simulink library "Adaptive_library"  (R2016b)
settings: Solver=ode45  StartTime=0.0  StopTime=10.0  RelTol=1e-3  EnableMultiTasking=on
undefined symbols (not defined in the file or in its folder): functionType
libraries: Adaptive_library x7, vrlib x2, dspinverses x2
settings Model: Creator=jinkale  LastModifiedBy=dell
settings DataIOCC: LimitDataPoints=on  SaveFormat=Array
settings OptimizationCC: LifeSpan=inf
settings DebuggingCC: SFUnexpectedBacktrackingDiag=warning  SFNoUnconditionalDefaultTransitionDiag=warning  SFExecutionAtInitializationDiag=none
settings HardwareCC: ProdBitPerPointer=32  ProdBitPerSizeT=32  ProdBitPerPtrDiffT=32  ProdLargestAtomicFloat=None  ProdIntDivRoundTo=Undefined  ProdEndianess=Unspecified  ProdWordSize=32  ProdHWDeviceType=32-bit Generic
settings ModelReferenceCC: PropagateSignalLabelsOutOfModel=off
settings GRTTargetCC: TargetLangStandard=C89/C90 (ANSI)  GeneratePreprocessorConditionals=Disable all
settings ConfigComp: CovMetricSettings=dw  CovHtmlReporting=on  CovSaveCumulativeToWorkspaceVar=on  CovSaveSingleToWorkspaceVar=on  CovExternalEMLEnable=off

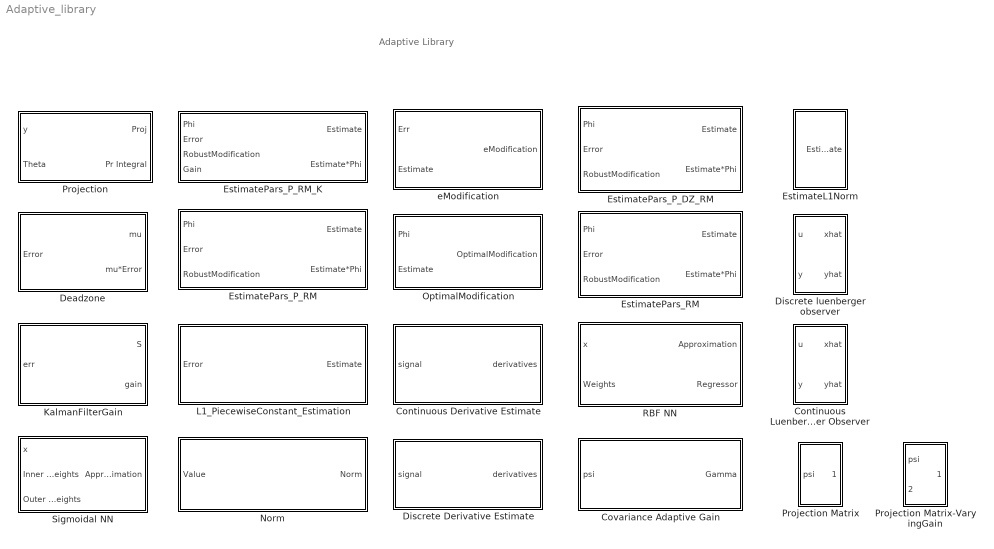
== system Adaptive_library ==
  note: Adaptive Library
  Continuous Derivative Estimate : Subsystem  mask{N=1, poles=[-300,-350], x0=0, satmax=10, satmin=-10}
      mask prompts: N "Derivative order"; poles "Observer poles"; x0 "Initial conditions"; satmax "Maximum saturation"; satmin "Minimum saturation"
      mask help:
      | % Name: Continuous Derivative Estimate
      | % Author: Alessio Russo - russo.alessio890@gmail.com
      | % Last update: 2/12/2016
      | % INPUTS
      | %      -signal: signal to differentiate
      | % OUTPUTS:
      | %      -derivatives: derivatives of signal
      |
      | Derivative order: up to which order we should estimate the derivative of signal
      | Observer poles: poles of the observer. Higher in absolute value-> faster. But there is peaking phenomena
      | Saturation: saturation on the signal derivatives
      mask init:
      | N=N+1;
      | A = [zeros(N-1,1), eye(N-1); zeros(1, N)];
      | B = zeros(N,1);
      | C = [1, zeros(1,N-1)];
      | D = 0;
      | 
      | L = place(A', C', poles)';
  "Continuous Luenberger Observer " : Subsystem  mask{A=0, B=0, C=0, D=0, L=0, x0=0, satmax=10, satmin=-10}
      mask prompts: L "Observer gain"; x0 "Initial condition"; satmax "Max saturation"; satmin "Min saturation"
      mask help:
      | % Name: Continuous Luenberger Observer
      | % Author: Alessio Russo - russo.alessio890@gmail.com
      | % Last update: 2/12/2016
      | % INPUTS
      | %      -u: input signal of the plant to observe
      | %      -y: output signal of the plant to observe
      | % OUTPUTS:
      | %      -xhat: estimated state of the plant
      | %      -yhat: estimated output of the plant
      |
      |
      | Continuous luenberger observer. The saturation block saturates the states.
      mask DialogControl Container3 Prompt: Parameters
  Covariance Adaptive Gain : Subsystem  mask{Gamma0=1, alpha1=1, alpha2=1, Kalpha1=1}
      mask prompts: Gamma0 "Initial condition"
      mask help:
      | % Name: Covariance Adaptive Gain
      | % Author: Alessio Russo - russo.alessio890@gmail.com
      | % Last update: 2/12/2016
      | % INPUTS
      | %      -psi: input feature psi(x)
      | % OUTPUTS:
      | %      -Gamma: adaptive gain
      |
      | Initial condition - Gamma0: positive definite diagonal matrix which defines the initial values for the adaptive gian.
      | Forgetting factor - Alpha1: positive definite diagonal matrix which defines the forgetting factor.
      | Excitation gain - Alpha2: positive definite diagonla matrix that defines the gain of the excitation
      | Maximum gain bound - Kalpha1 : defines the maximum bound of the inf norm of gamma
      |
      |
      | Equation:
      |
      | \dot{Gamma} = alpha1*Gamma- alpha2* Gamma*psi*psi^T *Gamma
      mask init:
      | if (Kalpha1 <= 0 || isscalar(Kalpha1)==0)
      |     error('Kalpha1 should be a scalar number greater than 0.')
      | end
      | 
      | if (isdiag(Gamma0)==0 || isdiag(alpha1)==0 || isdiag(alpha2)==0)
      |     error('One of the matrices is not diagonal.')
      | end
      | %the second value that chol returns is whether a matrix is positive
      | %definite (0) or not (1)
      | [~,p1] = chol(Gamma0);
      | [~,p2] = chol(alpha1);
      | [~,p3] = chol(alpha2);
      | 
      | if (p1 > 0)
      |     error('Gamma0 is not positive definite.')
      | end
      | if (p2 > 0)
      |     error('alpha1 is not positive definite')
      | end
      | 
      | if(p3 > 0)
      |     error('alpha2 is not positive definite')
      | end
  Deadzone : Subsystem  mask{delta=0.5, e0=1, Weight=1}
      mask prompts: delta "delta ( 0 < delta < 1)"; e0 "e0 ( e0 >0 )"
      mask help:
      | % Name: Deadzone with lipschitz modification
      | % Author: Alessio Russo - russo.alessio890@gmail.com
      | % Last update: 2/12/2016
      | % INPUTS
      | %      -Error: error between reference and plant
      | % OUTPUTS:
      | %      -mu: calculates mu(||Error||)
      | %      -mu*Error: claculates mu(||Error||)*Error
      |
      |
      | Implements the lipschitz-continuous version of the deadzone.
      |
      | mu(Error) = max(0, min (1, (||Error|- delta*e0)/((1-delta)*e0)));
      |
      | 0 < delta < 1
      | e0 > 0
      mask init:
      | if (e0<=0)
      |     error('e0 should be  greater than 0.')
      | end
      | 
      | if (delta <= 0 || delta >= 1)
      |     error('delta should lay in (0,1).');
      | end
  Discrete Derivative Estimate : Subsystem  mask{N=1, poles=[0.05,0.01], x0=0, ts=0.01, satmax=10, satmin=-10}
      mask prompts: N "Derivative order"; poles "Observer poles"; x0 "Initial conditions"; ts "Sampling time"; satmax "Maximum saturation"; satmin "Minimum saturation"
      mask help:
      | % Name: Discrete  Derivative Estimate
      | % Author: Alessio Russo - russo.alessio890@gmail.com
      | % Last update: 2/12/2016
      | % INPUTS
      | %      -signal: signal to differentiate
      | % OUTPUTS:
      | %      -derivatives: derivatives of signal
      |
      | Derivative order: up to which order we should estimate the derivative of signal
      | Observer poles: poles of the observer. Lower in absolute value-> faster. But there is peaking phenomena
      | Saturation: saturation on the signal derivatives
      mask init:
      | N=N+1;
      | A = [zeros(N-1,1), eye(N-1); zeros(1, N)];
      | B = zeros(N,1);
      | C = [1, zeros(1,N-1)];
      | D = 0;
      | 
      | A = (eye(N)+0.5*A*ts)*inv(eye(N)-0.5*A*ts);
      | L = place(A', C', poles)';
  Discrete luenberger observer : Subsystem  mask{A=0, B=0, C=0, D=0, L=0, x0=0, ts=0.1, satmax=10, satmin=-10}
      mask prompts: L "Observer gain"; x0 "Initial condition"; ts "Sampling time"; satmax "Maximum saturation"; satmin "Minimum saturation"
      mask help:
      | % Name: Discrete Luenberger Observer
      | % Author: Alessio Russo - russo.alessio890@gmail.com
      | % Last update: 2/12/2016
      | % INPUTS
      | %      -u: input signal of the plant to observe
      | %      -y: output signal of the plant to observe
      | % OUTPUTS:
      | %      -xhat: estimated state of the plant
      | %      -yhat: estimated output of the plant
      |
      |
      | Discrete luenberger observer. The saturation block saturates the states.
  EstimateL1Norm : Subsystem  mask{A=0, B=0, C=0, D=0, x0=0, df=100}
      mask prompts: x0 "X0 (Initial conditions)"; df "Derivative Frequency"
      mask help:
      | % Name: EstimateL1Norm
      | % Author: Alessio Russo - russo.alessio890@gmail.com
      | % Last update: 2/12/2016
      |
      |
      | BLOCK NOT COMPLETED! The output should be the l1 norm estimate of a linear SISO system
  EstimatePars_P_DZ_RM : Subsystem  mask{Gamma=100, P=0, B=0, EpsilonTheta=0.1, Prmax=1, Center=0, Pr0=0, delta=0.5, e0=1}
      mask prompts: EpsilonTheta "Epsilon"; Prmax "Bound (radius of the ball)"; Center "Center (of the ball)"; Pr0 "Initialization of the integral"; delta "delta ( 0 < delta < 1)"; e0 "e0 ( e0 >0 )"
      mask help:
      | % Name: EstimatePars_P_DZ_RM
      | % Author: Alessio Russo - russo.alessio890@gmail.com
      | % Last update: 2/12/2016
      | % INPUTS
      | %      -Phi: input feature phi(x)
      | %      -Error: error signal
      | %      -RobustModification: any additive robust modification can be included in this port
      | % OUTPUTS:
      | %      -Estimate: uncertainty estimate
      | %      -Estimate*Phi: uncertainty times the input feature
      |
      |
      | Used in conjuction with the projection operator and the lipschitz version of the deadzone,
      | implemented as follows:
      |
      | mu(e) = max(0, min (1, (||e|- delta*e0)/((1-delta)*e0)));
      |
      | 0 < delta < 1
      | e0 > 0
      mask init:
      | Pb=P*B;
      | 
      | if (e0<=0)
      |     error('e0 should be  greater than 0.')
      | end
      | 
      | if (delta <= 0 || delta >= 1)
      |     error('delta should lay in (0,1).');
      | end
  EstimatePars_P_RM : Subsystem  mask{Gamma=1, P=0, B=0, EpsilonTheta=0.1, Prmax=1, Center=0, Pr0=0}
      mask prompts: EpsilonTheta "Epsilon"; Prmax "Bound (radius of the ball)"; Center "Center (of the ball)"; Pr0 "Initialization of the integral"
      mask help:
      | % Name: EstimatePars_P_RM
      | % Author: Alessio Russo - russo.alessio890@gmail.com
      | % Last update: 2/12/2016
      | % INPUTS
      | %      -Phi: input feature phi(x)
      | %      -Error: error signal
      | %      -RobustModification: any additive robust modification can be included in this port
      | % OUTPUTS:
      | %      -Estimate: uncertainty estimate
      | %      -Estimate*Phi: uncertainty times the input feature
      |
      | The block implements the projection operator
      mask init:
      | Pb=P*B;
  EstimatePars_P_RM_K : Subsystem  mask{P=0, B=0, EpsilonTheta=0.1, Prmax=1, Center=0, Pr0=0}
      mask prompts: EpsilonTheta "Epsilon"; Prmax "Bound (radius of the ball)"; Center "Center (of the ball)"; Pr0 "Initialization of the integral"
      mask help:
      | % Name: EstimatePars_P_RM_K
      | % Author: Alessio Russo - russo.alessio890@gmail.com
      | % Last update: 2/12/2016
      | % INPUTS
      | %      -Phi: input feature phi(x)
      | %      -Error: error signal
      | %      -RobustModification: any additive robust modification can be included in this port
      | %      -Gain: adaptive gain (external)
      | % OUTPUTS:
      | %      -Estimate: uncertainty estimate
      | %      -Estimate*Phi: uncertainty times the input feature
      |
      | The block implements the projection operator
      mask init:
      | Pb=P*B;
  EstimatePars_RM : Subsystem  mask{Gamma=0, x0=0, P=0, B=0}
      mask prompts: x0 "InitialValue"
      mask help:
      | % Name: EstimatePars_RM
      | % Author: Alessio Russo - russo.alessio890@gmail.com
      | % Last update: 2/12/2016
      | % INPUTS
      | %      -Phi: input feature phi(x)
      | %      -Error: error signal
      | %      -RobustModification: any additive robust modification can be included in this port
      | % OUTPUTS:
      | %      -Estimate: uncertainty estimate
      | %      -Estimate*Phi: uncertainty times the input feature
      mask init:
      | Pb=P*B;
  KalmanFilterGain : Subsystem  mask{Q=1, R=1, S0=1, sigma=1}
      mask help:
      | % Name:  KalmanFilterGain
      | % Author: Alessio Russo - russo.alessio890@gmail.com
      | % Last update: 2/12/2016
      | % INPUTS
      | %      -err: error signal
      | % OUTPUTS:
      | %      -S: matrix S(t) used to calculate the adaptive gain
      | %      -gain: adaptive gain Gamma
      |
      | Gamma is calculated as follows
      |
      | Gamma = S*inv(R)
      |
      | where \dot{S} = -sigma *||e|| *S*inv(R)*S+Q
      |
      | and, Q,R are symmetric positive definite matrices (fixed). S0 defines the initial condition of S(t).
  L1_PiecewiseConstant_Estimation : Subsystem  mask{Bm=1, Bum=0, Ts=1, Am=-1, gamma=1, x0=0, satmax=inf, satmin=-inf}
      mask prompts: Bm "Bm (Matched)"; Bum "Bum (Unmatched)"; Ts "Sampling Time"; Am "Am (reference matrix of dynamics)"; x0 "Initial Value"; satmax "Max Saturation"; satmin "Min Saturation"
      mask help:
      | % Name: L1 Piecewise-constant adaptive law
      | % Author: Alessio Russo - russo.alessio890@gmail.com
      | % Last update: 2/12/2016
      | % INPUTS
      | %      -error: error signal
      | % OUTPUTS:
      | %      -estimate: uncertainty estimate
      |
      | The output of the block is the estimate that needs to be cancelled.
      mask init:
      | if (Ts<=0)
      |     error('Sampling time should be  greater than 0.')
      | end
      | 
      | if (gamma<=0)
      |     error('Gamma should be  greater than 0.')
      | end
      | 
      | if (sum(real(eig(Am))>=0))
      |     error('Am should be Hurwitz.');
      | end
      | 
      | 
      | mu = exp(Am*Ts);
      | if (isscalar(Bm)==1 || (size(Bm,1)==size(Bm,2)))
      |     B=Bm;
      | else
      |     B = [Bm, Bum];
      | end
      | PHIinv = inv(inv(Am)* ( exp(Am*Ts)- eye(size(Am,1)))*B);
  Norm : Subsystem
      mask help:
      | % Name: Norm
      | % Author: Alessio Russo - russo.alessio890@gmail.com
      | % Last update: 2/12/2016
      | % INPUTS
      | %      -Value: vector input
      | % OUTPUTS:
      | %      -Norm: euclidean norm of Value
  OptimalModification : Subsystem  mask{sigma=1, P=0, B=0, Am=0}
      mask help:
      | % Name: optimal modification
      | % Author: Alessio Russo - russo.alessio890@gmail.com
      | % Last update: 2/12/2016
      | % INPUTS
      | %      -phi: phi(x) , input feature
      | %      -estimate: uncertainty estimate
      | % OUTPUTS:
      | %      -optimal modification: gives as output the optimal modification that should be added to the adaptive law
      mask init:
      | OptConst = B'*P*inv(Am)*B;
  Projection : Subsystem  mask{EpsilonTheta=0.3, Prmax=0.5, Center=0, Pr0=0.1}
      mask prompts: EpsilonTheta "Epsilon"; Prmax "Bound (radius of the ball)"; Center "Center (of the ball)"; Pr0 "Initialization of integral"
      mask help:
      | % Name: Projection Operator with center modification
      | % Author: Alessio Russo - russo.alessio890@gmail.com
      | % Last update: 2/12/2016
      | % INPUTS
      | %      -y: value to project
      | %      -theta: current value of the estimate
      | % OUTPUTS:
      | %      -Proj: calculates Proj(theta,y)
      | %      -Pr Integral: integrates Proj(theta;y)
      |
      | Computes projection of the signal and safely integrate it.
      | Works both for scalar and vector signals.
      | It considers the parameter set as a ball at the setted center and radius.
      |
      | Epsilon defines when the projection operator starts to operate.
      mask init:
      | Thetamax = (Prmax) / sqrt(EpsilonTheta+1);
  Projection Matrix : Subsystem  mask{Gamma=1}
      mask prompts: Gamma "Adaptive gain matrix"
      mask help:
      | % Name: Projection Matrix
      | % Author: Alessio Russo - russo.alessio890@gmail.com
      | % Last update: 26/12/2016
      | % INPUTS
      | %      -psi: input feature psi(x)
      | % OUTPUTS:
      | %      -Proj: projection matrix
      |
      | Outputs a matrix that projects any vector on the null space of psi. Gamma is a positive definite symmetric matrix.
      |
      | The matrix is calculated based on the following law
      |
      | I- A(A^TA)^(-1)A^T, where A = Gamma*psi
  Projection Matrix-VaryingGain : Subsystem
      mask help:
      | % Name: Projection Matrix-VaryingGain
      | % Author: Alessio Russo - russo.alessio890@gmail.com
      | % Last update: 26/12/2016
      | % INPUTS
      | %      -psi: input feature psi(x)
      | %      -Gamma: definite positive symmetric matrix
      | % OUTPUTS:
      | %      -Proj: projection matrix
      |
      | Outputs a matrix that projects any vector on the null space of psi. Gamma is a positive definite symmetric matrix.
      |
      | The matrix is calculated based on the following law
      |
      | I- A(A^TA)^(-1)A^T, where A = Gamma*psi
  RBF NN : Subsystem  mask{Mean=0, Variance=0}
      mask help:
      | % Name: RBF NN
      | % Author: Alessio Russo - russo.alessio890@gmail.com
      | % Last update: 2/12/2016
      | % INPUTS
      | %      -x: input feature
      | %      -Weights: weights of the GMM
      | % OUTPUTS:
      | %      -Approximation: output of the GMM NN
      | %      -Regressor: vector of the basis functions output
      |
      | This RBF block implement the GMM (gaussian mixture model) which is just a linear combination of gaussian functions.
      | Mean is  a vector containing the center of the gaussians functions. Variance is a vector defining
      | the variance of each gaussian.
      |
      | y(x) = W * [exp(-Variance * (x-Mean)^2)]
  Sigmoidal NN : Subsystem  mask{rf=Logistic sigmoid}
      mask prompts: rf "Ridge Function"
      mask help:
      | % Name: Sigmoidal NN
      | % Author: Alessio Russo - russo.alessio890@gmail.com
      | % Last update: 2/12/2016
      | % INPUTS
      | %      -x: input feature
      | %      -Inner Weights: weights matrix of the hidden layer
      | %      - Outer Weight: weights matrix of the output layer
      | % OUTPUTS:
      | %      -Approximation: output of the NN
      |
      | Sigmoidal NN. The logistic or hyperbolic tangent functions can be used
      mask init:
      | switch rf
      |     case 'Logistic sigmoid'
      |         FunctionType = -1;
      |     case 'Hyperbolic tangent'
      |         FunctionType = 1;
      | end
      mask TypeOptions rf: Logistic sigmoid | Hyperbolic tangent
  eModification : Subsystem  mask{sigma=0, P=0, B=0}
      mask help:
      | % Name: e modification
      | % Author: Alessio Russo - russo.alessio890@gmail.com
      | % Last update: 2/12/2016
      | % INPUTS
      | %      -err: error signal
      | %      -estimate: uncertainty estimate
      | % OUTPUTS:
      | %      -e modification: gives as output sigma*||e(t)^TPB||*estimate
      |
      | Givent the values for sigma, P, B calculates sigma*||e(t)^TPB||*estimate
      mask init:
      | Pb=P*B;

== system Adaptive_library/Continuous Derivative Estimate ==
  signal : Inport
  Continuous Luenberger Observer1 : Adaptive_library/Continuous Luenberger Observer  A=A  B=B  C=C  D=D  L=L  x0=x0  satmax=satmax  satmin=satmin
  Ground : Ground
  Terminator : Terminator
  derivatives : Outport
  wires:
  Continuous Luenberger Observer1/2 -> Terminator/1
  Continuous Luenberger Observer1/1 -> derivatives/1
  Ground/1 -> Continuous Luenberger Observer1/1
  signal/1 -> Continuous Luenberger Observer1/2

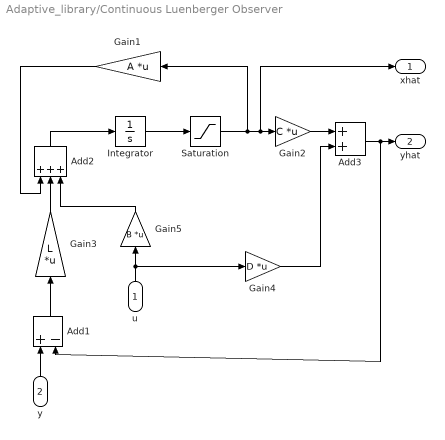
== system Adaptive_library/Continuous Luenberger Observer  ==
  u : Inport
  y : Inport  Port=2
  Add1 : Sum  Inputs=+-
  Add2 : Sum  Inputs=+++
  Add3 : Sum
  Gain1 : Gain  Gain=A  Multiplication=Matrix(K*u)
  Gain2 : Gain  Gain=C  Multiplication=Matrix(K*u)
  Gain3 : Gain  Gain=L  Multiplication=Matrix(K*u)
  Gain4 : Gain  Gain=D  Multiplication=Matrix(K*u)
  Gain5 : Gain  Gain=B  Multiplication=Matrix(K*u)
  Integrator : Integrator  InitialCondition=x0
  Saturation : Saturate  UpperLimit=satmax  LowerLimit=satmin
  xhat : Outport
  yhat : Outport  Port=2
  wires:
  Gain3/1 -> Add2/2
  Gain1/1 -> Add2/1
  Integrator/1 -> Saturation/1
  Add2/1 -> Integrator/1
  y/1 -> Add1/1
  Add1/1 -> Gain3/1
  Gain5/1 -> Add2/3
  Gain2/1 -> Add3/1
  Gain4/1 -> Add3/2
  u/1 -> Gain4/1, Gain5/1
  Add3/1 -> Add1/2, yhat/1
  Saturation/1 -> xhat/1, Gain2/1, Gain1/1

== system Adaptive_library/Covariance Adaptive Gain ==
  psi : Inport
  Integrator : Integrator  InitialCondition=Gamma0
  Math Function : Math  Operator=transpose  SaturateOnIntegerOverflow=on
  Math Function1 : Math  Operator=transpose  SaturateOnIntegerOverflow=on
  Product : Product  Multiplication=Matrix(*)
  Product1 : Product  Multiplication=Matrix(*)
  Subsystem : Subsystem
  Subtract : Sum  Inputs=+-
  alpha2 : Gain  Gain=alpha2  Multiplication=Matrix(K*u)
  Gamma : Outport
  wires:
  Math Function/1 -> Product/1
  Subtract/1 -> Integrator/1
  Integrator/1 -> Gamma/1, Product/2, Subsystem/1(Gamma)
  alpha2/1 -> Subtract/2
  Product/1 -> Product1/2, Math Function1/1
  psi/1 -> Math Function/1
  Math Function1/1 -> Product1/1
  Product1/1 -> alpha2/1
  Subsystem/1(alpha1*Gamma) -> Subtract/1

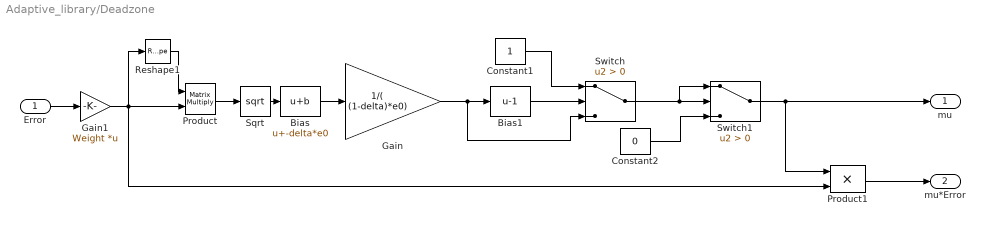
== system Adaptive_library/Deadzone ==
  Error : Inport
  Bias : Bias  Bias=-delta*e0
  Bias1 : Bias  Bias=-1
  Constant1 : Constant
  Constant2 : Constant  Value=0
  Gain : Gain  Gain=1/( (1-delta)*e0)
  Gain1 : Gain  Gain=Weight  Multiplication=Matrix(K*u)
  Product : Product  Multiplication=Matrix(*)
  Product1 : Product
  Reshape1 : Reshape  OutputDimensionality=Row vector (2-D)
  Sqrt : Sqrt  SaturateOnIntegerOverflow=on
  Switch : Switch  Criteria=u2 > Threshold
  Switch1 : Switch  Criteria=u2 > Threshold
  mu : Outport
  mu*Error : Outport  Port=2
  wires:
  Bias/1 -> Gain/1
  Gain/1 -> Switch/3, Bias1/1
  Bias1/1 -> Switch/2
  Constant1/1 -> Switch/1
  Switch/1 -> Switch1/1, Switch1/2
  Constant2/1 -> Switch1/3
  Switch1/1 -> Product1/1, mu/1
  Reshape1/1 -> Product/1
  Sqrt/1 -> Bias/1
  Product/1 -> Sqrt/1
  Product1/1 -> mu*Error/1
  Error/1 -> Gain1/1
  Gain1/1 -> Reshape1/1, Product1/2, Product/2

== system Adaptive_library/Discrete Derivative Estimate ==
  signal : Inport
  Discrete luenberger observer1 : Adaptive_library/Discrete luenberger observer  A=A  B=B  C=C  D=D  L=L  x0=x0  ts=ts  satmax=satmax  satmin=satmin
  Ground : Ground
  Terminator : Terminator
  Zero-Order Hold : ZeroOrderHold  SampleTime=ts
  Zero-Order Hold1 : ZeroOrderHold  SampleTime=ts
  derivatives : Outport
  wires:
  Discrete luenberger observer1/1 -> Zero-Order Hold1/1
  Ground/1 -> Discrete luenberger observer1/1
  signal/1 -> Zero-Order Hold/1
  Discrete luenberger observer1/2 -> Terminator/1
  Zero-Order Hold/1 -> Discrete luenberger observer1/2
  Zero-Order Hold1/1 -> derivatives/1

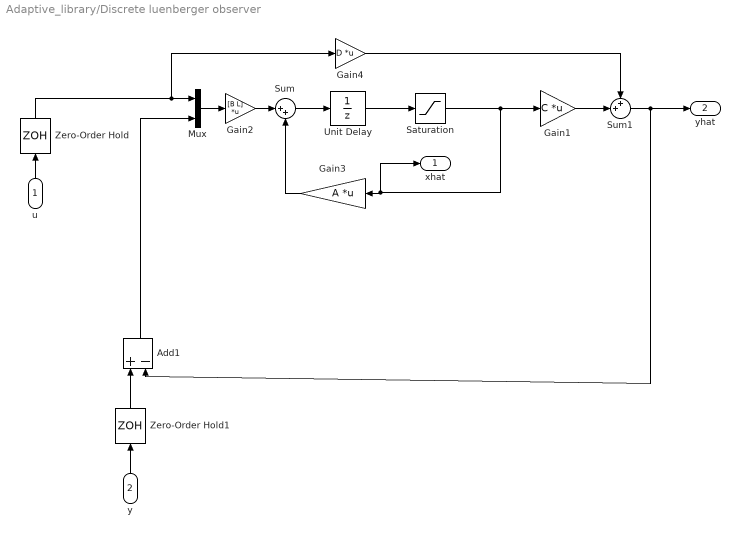
== system Adaptive_library/Discrete luenberger observer ==
  u : Inport
  y : Inport  Port=2
  Add1 : Sum  Inputs=+-
  Gain1 : Gain  Gain=C  Multiplication=Matrix(K*u)
  Gain2 : Gain  Gain=[B L]  Multiplication=Matrix(K*u)
  Gain3 : Gain  Gain=A  Multiplication=Matrix(K*u)
  Gain4 : Gain  Gain=D  Multiplication=Matrix(K*u)
  Mux : Mux  Inputs=2
  Saturation : Saturate  UpperLimit=satmax  LowerLimit=satmin
  Sum : Sum  Inputs=|++
  Sum1 : Sum  Inputs=++|
  Unit Delay : UnitDelay  InitialCondition=x0  SampleTime=ts
  Zero-Order Hold : ZeroOrderHold  SampleTime=ts
  Zero-Order Hold1 : ZeroOrderHold  SampleTime=ts
  xhat : Outport
  yhat : Outport  Port=2
  wires:
  Add1/1 -> Mux/2
  y/1 -> Zero-Order Hold1/1
  u/1 -> Zero-Order Hold/1
  Zero-Order Hold1/1 -> Add1/1
  Zero-Order Hold/1 -> Gain4/1, Mux/1
  Unit Delay/1 -> Saturation/1
  Mux/1 -> Gain2/1
  Gain2/1 -> Sum/1
  Sum/1 -> Unit Delay/1
  Gain3/1 -> Sum/2
  Gain1/1 -> Sum1/2
  Sum1/1 -> Add1/2, yhat/1
  Gain4/1 -> Sum1/1
  Saturation/1 -> Gain1/1, xhat/1, Gain3/1

== system Adaptive_library/EstimateL1Norm ==
  Abs : Abs
  Integrator : Integrator
  State-Space : StateSpace  A=A  B=B  C=C  D=D  X0=x0
  Step : Step  After=2*pi*df  SampleTime=0
  Transfer Fcn1 : TransferFcn  Numerator=[1 0]  Denominator=[1 2*pi*df]
  Estimate : Outport
  wires:
  State-Space/1 -> Abs/1
  Step/1 -> Transfer Fcn1/1
  Abs/1 -> Integrator/1
  Transfer Fcn1/1 -> State-Space/1
  Integrator/1 -> Estimate/1

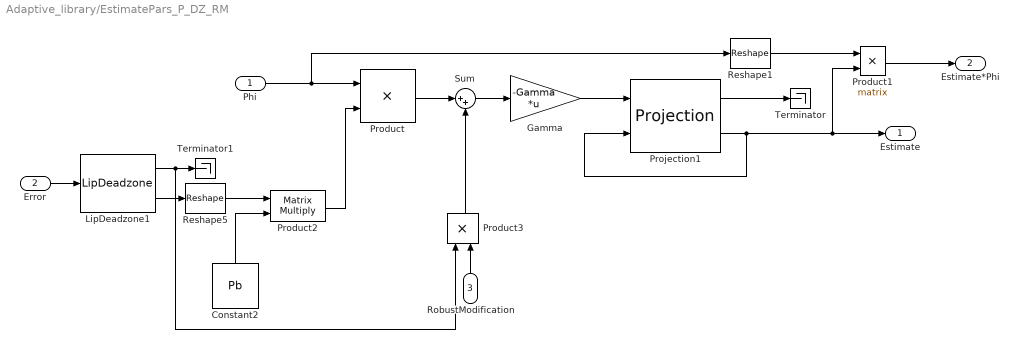
== system Adaptive_library/EstimatePars_P_DZ_RM ==
  Phi : Inport
  Error : Inport  Port=2
  RobustModification : Inport  Port=3
  Constant2 : Constant  Value=Pb
  Gamma : Gain  Gain=-Gamma  Multiplication=Matrix(K*u)
  LipDeadzone1 : Adaptive_library/LipDeadzone  delta=delta  e0=e0  Weight=1
  Product : Product  RndMeth=Zero
  Product1 : Product  Multiplication=Matrix(*)  RndMeth=Zero
  Product2 : Product  Multiplication=Matrix(*)  RndMeth=Zero
  Product3 : Product
  Projection1 : Adaptive_library/Projection  EpsilonTheta=EpsilonTheta  Prmax=Prmax  Center=Center  Pr0=Pr0
  Reshape1 : Reshape  OutputDimensionality=Row vector (2-D)
  Reshape5 : Reshape  OutputDimensionality=Row vector (2-D)
  Sum : Sum  Inputs=|++
  Terminator : Terminator
  Terminator1 : Terminator
  Estimate : Outport
  Estimate*Phi : Outport  Port=2
  wires:
  Gamma/1 -> Projection1/1
  Reshape5/1 -> Product2/1
  Constant2/1 -> Product2/2
  Projection1/2 -> Projection1/2, Estimate/1, Product1/2
  Projection1/1 -> Terminator/1
  Product2/1 -> Product/2
  Phi/1 -> Reshape1/1, Product/1
  Product1/1 -> Estimate*Phi/1
  LipDeadzone1/2 -> Reshape5/1
  LipDeadzone1/1 -> Product3/1, Terminator1/1
  Error/1 -> LipDeadzone1/1
  Sum/1 -> Gamma/1
  Product/1 -> Sum/1
  RobustModification/1 -> Product3/2
  Product3/1 -> Sum/2
  Reshape1/1 -> Product1/1

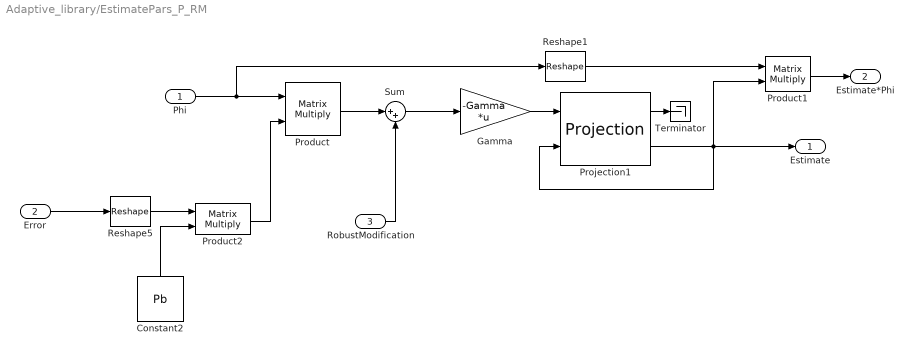
== system Adaptive_library/EstimatePars_P_RM ==
  Phi : Inport
  Error : Inport  Port=2
  RobustModification : Inport  Port=3
  Constant2 : Constant  Value=Pb
  Gamma : Gain  Gain=-Gamma  Multiplication=Matrix(K*u)
  Product : Product  Multiplication=Matrix(*)  RndMeth=Zero
  Product1 : Product  Multiplication=Matrix(*)  RndMeth=Zero
  Product2 : Product  Multiplication=Matrix(*)  RndMeth=Zero
  Projection1 : Adaptive_library/Projection  EpsilonTheta=EpsilonTheta  Prmax=Prmax  Center=Center  Pr0=Pr0
  Reshape1 : Reshape  OutputDimensionality=Row vector (2-D)
  Reshape5 : Reshape  OutputDimensionality=Row vector (2-D)
  Sum : Sum  Inputs=|++
  Terminator : Terminator
  Estimate : Outport
  Estimate*Phi : Outport  Port=2
  wires:
  Gamma/1 -> Projection1/1
  Reshape5/1 -> Product2/1
  Constant2/1 -> Product2/2
  Projection1/2 -> Projection1/2, Product1/2, Estimate/1
  Projection1/1 -> Terminator/1
  Product2/1 -> Product/2
  Phi/1 -> Reshape1/1, Product/1
  Product1/1 -> Estimate*Phi/1
  Error/1 -> Reshape5/1
  Sum/1 -> Gamma/1
  Product/1 -> Sum/1
  RobustModification/1 -> Sum/2
  Reshape1/1 -> Product1/1

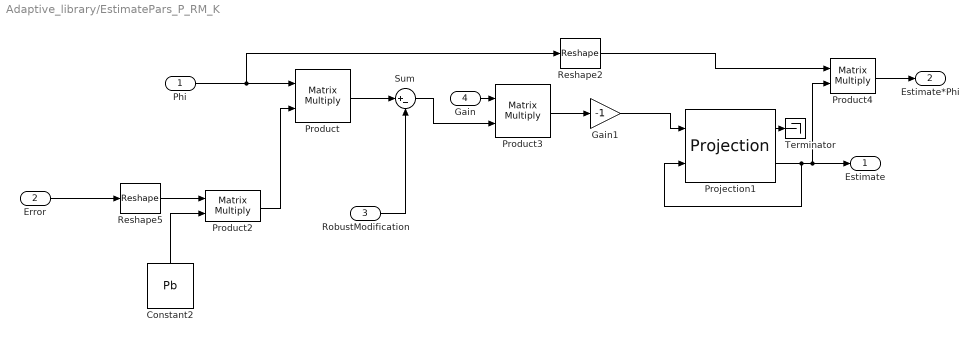
== system Adaptive_library/EstimatePars_P_RM_K ==
  Phi : Inport
  Error : Inport  Port=2
  RobustModification : Inport  Port=3
  Gain : Inport  Port=4
  Constant2 : Constant  Value=Pb
  Gain1 : Gain  Gain=-1
  Product{,2..4} (4 alike) : Product  Multiplication=Matrix(*)  RndMeth=Zero
  Projection1 : Adaptive_library/Projection  EpsilonTheta=EpsilonTheta  Prmax=Prmax  Center=Center  Pr0=Pr0
  Reshape2 : Reshape  OutputDimensionality=Row vector (2-D)
  Reshape5 : Reshape  OutputDimensionality=Row vector (2-D)
  Sum : Sum  Inputs=|+-
  Terminator : Terminator
  Estimate : Outport
  Estimate*Phi : Outport  Port=2
  wires:
  RobustModification/1 -> Sum/2
  Phi/1 -> Reshape2/1, Product/1
  Product2/1 -> Product/2
  Reshape5/1 -> Product2/1
  Constant2/1 -> Product2/2
  Product/1 -> Sum/1
  Error/1 -> Reshape5/1
  Product3/1 -> Gain1/1
  Projection1/2 -> Projection1/2, Product4/2, Estimate/1
  Projection1/1 -> Terminator/1
  Product4/1 -> Estimate*Phi/1
  Reshape2/1 -> Product4/1
  Gain1/1 -> Projection1/1
  Gain/1 -> Product3/1
  Sum/1 -> Product3/2

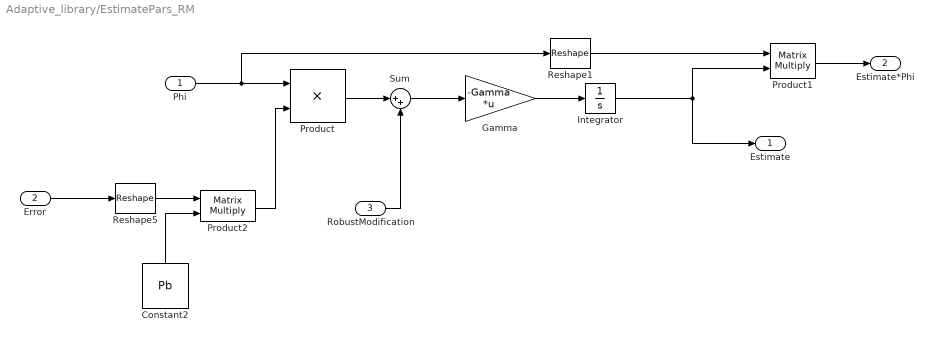
== system Adaptive_library/EstimatePars_RM ==
  Phi : Inport
  Error : Inport  Port=2
  RobustModification : Inport  Port=3
  Constant2 : Constant  Value=Pb
  Gamma : Gain  Gain=-Gamma  Multiplication=Matrix(K*u)
  Integrator : Integrator  InitialCondition=x0
  Product : Product  RndMeth=Zero
  Product1 : Product  Multiplication=Matrix(*)  RndMeth=Zero
  Product2 : Product  Multiplication=Matrix(*)  RndMeth=Zero
  Reshape1 : Reshape  OutputDimensionality=Row vector (2-D)
  Reshape5 : Reshape  OutputDimensionality=Row vector (2-D)
  Sum : Sum  Inputs=|++
  Estimate : Outport
  Estimate*Phi : Outport  Port=2
  wires:
  Gamma/1 -> Integrator/1
  Reshape5/1 -> Product2/1
  Constant2/1 -> Product2/2
  Integrator/1 -> Estimate/1, Product1/2
  Product2/1 -> Product/2
  Phi/1 -> Reshape1/1, Product/1
  Product1/1 -> Estimate*Phi/1
  Error/1 -> Reshape5/1
  Sum/1 -> Gamma/1
  Product/1 -> Sum/1
  RobustModification/1 -> Sum/2
  Reshape1/1 -> Product1/1

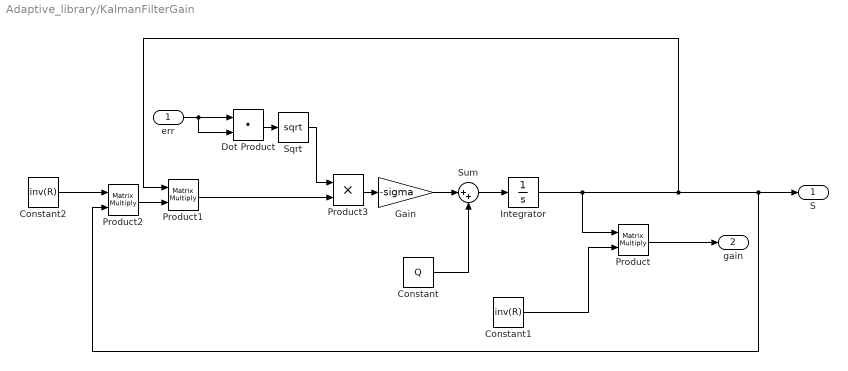
== system Adaptive_library/KalmanFilterGain ==
  err : Inport
  Constant : Constant  Value=Q
  Constant1 : Constant  Value=inv(R)
  Constant2 : Constant  Value=inv(R)
  Dot Product : DotProduct  InputSameDT=on  OutDataTypeStr=Inherit: Inherit via internal rule
  Gain : Gain  Gain=-sigma
  Integrator : Integrator  InitialCondition=S0
  Product : Product  Multiplication=Matrix(*)
  Product1 : Product  Multiplication=Matrix(*)
  Product2 : Product  Multiplication=Matrix(*)
  Product3 : Product
  Sqrt : Sqrt  SaturateOnIntegerOverflow=on
  Sum : Sum  Inputs=|++
  S : Outport
  gain : Outport  Port=2
  wires:
  Product3/1 -> Gain/1
  Constant1/1 -> Product/2
  Sum/1 -> Integrator/1
  Product1/1 -> Product3/2
  Integrator/1 -> Product/1, Product2/2, S/1, Product1/1
  Constant/1 -> Sum/2
  Constant2/1 -> Product2/1
  Product/1 -> gain/1
  Gain/1 -> Sum/1
  Product2/1 -> Product1/2
  err/1 -> Dot Product/2, Dot Product/1
  Dot Product/1 -> Sqrt/1
  Sqrt/1 -> Product3/1

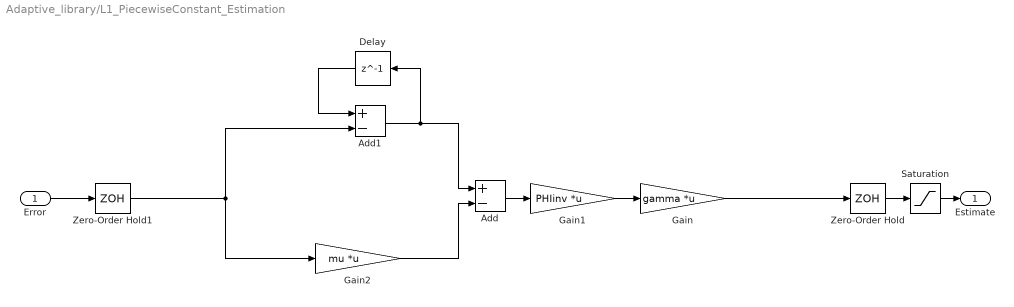
== system Adaptive_library/L1_PiecewiseConstant_Estimation ==
  Error : Inport
  Add : Sum  Inputs=+-
  Add1 : Sum  Inputs=+-
  Delay : Delay  DelayLength=1  InitialCondition=0  SampleTime=Ts
  Gain : Gain  Gain=gamma  Multiplication=Matrix(K*u)
  Gain1 : Gain  Gain=PHIinv  Multiplication=Matrix(K*u)
  Gain2 : Gain  Gain=mu  Multiplication=Matrix(K*u)
  Saturation : Saturate  UpperLimit=satmax  LowerLimit=satmin
  Zero-Order Hold : ZeroOrderHold  SampleTime=Ts
  Zero-Order Hold1 : ZeroOrderHold  SampleTime=Ts
  Estimate : Outport
  wires:
  Add/1 -> Gain1/1
  Zero-Order Hold/1 -> Saturation/1
  Error/1 -> Zero-Order Hold1/1
  Zero-Order Hold1/1 -> Gain2/1, Add1/2
  Gain2/1 -> Add/2
  Delay/1 -> Add1/1
  Add1/1 -> Delay/1, Add/1
  Gain1/1 -> Gain/1
  Saturation/1 -> Estimate/1
  Gain/1 -> Zero-Order Hold/1

== system Adaptive_library/Norm ==
  Value : Inport
  Dot Product : DotProduct  InputSameDT=on  OutDataTypeStr=Inherit: Inherit via internal rule
  Sqrt : Sqrt  SaturateOnIntegerOverflow=on
  Norm : Outport
  wires:
  Dot Product/1 -> Sqrt/1
  Value/1 -> Dot Product/2, Dot Product/1
  Sqrt/1 -> Norm/1

== system Adaptive_library/OptimalModification ==
  Phi : Inport
  Estimate : Inport  Port=2
  Constant : Constant  Value=OptConst
  Gain : Gain  Gain=sigma
  Product1 : Product  Multiplication=Matrix(*)  RndMeth=Zero
  Product2 : Product  Multiplication=Matrix(*)  RndMeth=Zero
  Product3 : Product  Multiplication=Matrix(*)  RndMeth=Zero
  Reshape5 : Reshape  OutputDimensionality=Row vector (2-D)
  OptimalModification : Outport
  wires:
  Phi/1 -> Product2/1, Reshape5/1
  Reshape5/1 -> Product2/2
  Gain/1 -> OptimalModification/1
  Constant/1 -> Product1/2
  Estimate/1 -> Product1/1
  Product2/1 -> Product3/1
  Product1/1 -> Product3/2
  Product3/1 -> Gain/1

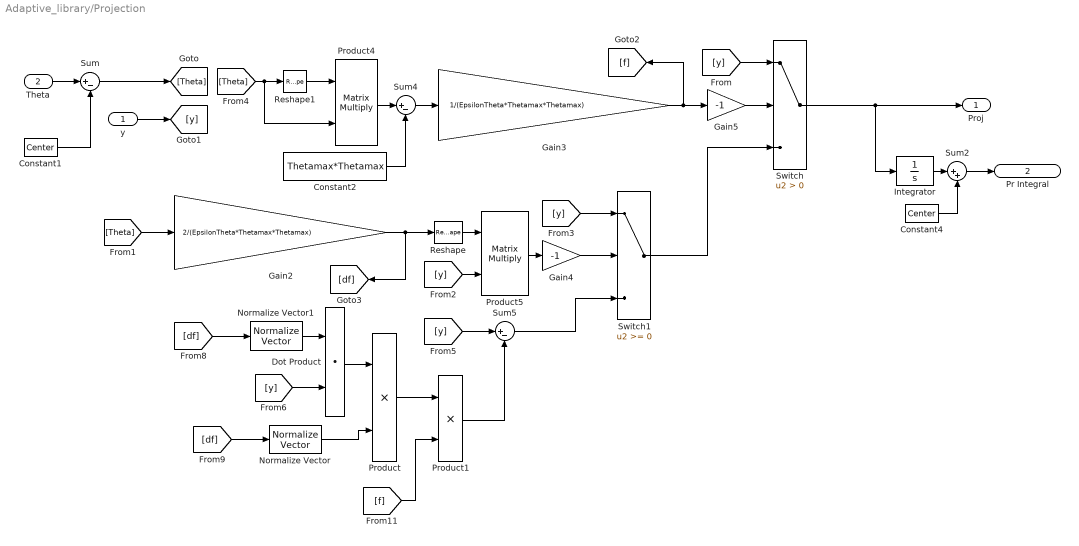
== system Adaptive_library/Projection ==
  y : Inport
  Theta : Inport  Port=2
  Constant1 : Constant  Value=Center
  Constant2 : Constant  Value=Thetamax*Thetamax
  Constant4 : Constant  Value=Center
  Dot Product : DotProduct  InputSameDT=on  OutDataTypeStr=Inherit: Inherit via internal rule
  Gain2 : Gain  Gain=2/(EpsilonTheta*Thetamax*Thetamax)
  Gain3 : Gain  Gain=1/(EpsilonTheta*Thetamax*Thetamax)
  Gain4 : Gain  Gain=-1
  Gain5 : Gain  Gain=-1
  Integrator : Integrator  InitialCondition=Pr0-Center  LimitOutput=on  UpperSaturationLimit=Prmax  LowerSaturationLimit=-Prmax
  Normalize Vector : vrlib/Utilities/Normalize Vector  maxzero=0
  Normalize Vector1 : vrlib/Utilities/Normalize Vector  maxzero=0
  Product : Product  RndMeth=Zero
  Product1 : Product  RndMeth=Zero
  Product4 : Product  Multiplication=Matrix(*)  RndMeth=Zero
  Product5 : Product  Multiplication=Matrix(*)  RndMeth=Zero
  Reshape : Reshape  OutputDimensionality=Row vector (2-D)
  Reshape1 : Reshape  OutputDimensionality=Row vector (2-D)
  Sum : Sum  Inputs=|+-
  Sum2 : Sum  Inputs=|++
  Sum4 : Sum  Inputs=|+-
  Sum5 : Sum  Inputs=|+-
  Switch : Switch  Criteria=u2 > Threshold
  Switch1 : Switch
  Proj : Outport
  Pr Integral : Outport  Port=2
  wires:
  Gain5/1 -> Switch/2
  Sum5/1 -> Switch1/3
  [y] -> Sum5/1
  Switch1/1 -> Switch/3
  [Theta] -> Gain2/1
  [y] -> Switch1/1
  Gain4/1 -> Switch1/2
  Product5/1 -> Gain4/1
  [y] -> Product5/2
  [y] -> Switch/1
  Gain3/1 -> [f], Gain5/1
  Sum4/1 -> Gain3/1
  Constant2/1 -> Sum4/2
  Product4/1 -> Sum4/1
  [Theta] -> Reshape1/1, Product4/2
  Gain2/1 -> Reshape/1, [df]
  Reshape/1 -> Product5/1
  Reshape1/1 -> Product4/1
  [df] -> Normalize Vector1/1
  [df] -> Normalize Vector/1
  Normalize Vector1/1 -> Dot Product/1
  [y] -> Dot Product/2
  Dot Product/1 -> Product/1
  Normalize Vector/1 -> Product/2
  Product/1 -> Product1/1
  [f] -> Product1/2
  Product1/1 -> Sum5/2
  Sum/1 -> [Theta]
  Theta/1 -> Sum/1
  Switch/1 -> Proj/1, Integrator/1
  Constant1/1 -> Sum/2
  y/1 -> [y]
  Sum2/1 -> Pr Integral/1
  Integrator/1 -> Sum2/1
  Constant4/1 -> Sum2/2

== system Adaptive_library/Projection Matrix ==
  psi : Inport
  " LU Inverse" : dspinverses/ LU Inverse
  Add : Sum  Inputs=+-
  Gain : Gain  Gain=Gamma  Multiplication=Matrix(K*u)
  Interpreted MATLAB Function : MATLABFcn  MATLABFcn=eye(length(u))  Output1D=off
  Math Function : Math  Operator=transpose  SaturateOnIntegerOverflow=on
  Product : Product  Multiplication=Matrix(*)
  Product1 : Product  Multiplication=Matrix(*)
  Product2 : Product  Multiplication=Matrix(*)
  Proj : Outport
  wires:
  Product2/1 -> Add/2
  Math Function/1 -> Product2/2, Product1/1
  Gain/1 -> Product1/2, Math Function/1, Product/1
  Add/1 -> Proj/1
  Product/1 -> Product2/1
  Interpreted MATLAB Function/1 -> Add/1
  psi/1 -> Interpreted MATLAB Function/1, Gain/1
  Product1/1 -> " LU Inverse"/1
  " LU Inverse"/1 -> Product/2

== system Adaptive_library/Projection Matrix-VaryingGain ==
  psi : Inport
  Gamma : Inport  Port=2
  " LU Inverse" : dspinverses/ LU Inverse
  Add : Sum  Inputs=+-
  Interpreted MATLAB Function : MATLABFcn  MATLABFcn=eye(length(u))  Output1D=off
  Math Function : Math  Operator=transpose  SaturateOnIntegerOverflow=on
  Product{,1..3} (4 alike) : Product  Multiplication=Matrix(*)
  Proj : Outport
  wires:
  Product3/1 -> Add/2
  Math Function/1 -> Product3/2, Product1/1
  Product2/1 -> Product1/2, Math Function/1, Product/1
  Add/1 -> Proj/1
  Product/1 -> Product3/1
  Interpreted MATLAB Function/1 -> Add/1
  psi/1 -> Interpreted MATLAB Function/1, Product2/2
  Gamma/1 -> Product2/1
  Product1/1 -> " LU Inverse"/1
  " LU Inverse"/1 -> Product/2

== system Adaptive_library/RBF NN ==
  x : Inport
  Weights : Inport  Port=2
  Constant1 : Constant  Value=Mean
  Gain : Gain  Gain=-Variance
  Math Function : Math  SaturateOnIntegerOverflow=on
  Math Function1 : Math  Operator=square  SaturateOnIntegerOverflow=on
  Math Function2 : Math  Operator=transpose  SaturateOnIntegerOverflow=on
  Product : Product  Multiplication=Matrix(*)
  Sum : Sum  Inputs=|+-
  Approximation : Outport
  Regressor : Outport  Port=2
  wires:
  Gain/1 -> Math Function/1
  x/1 -> Sum/1
  Constant1/1 -> Sum/2
  Math Function2/1 -> Product/1
  Math Function1/1 -> Gain/1
  Sum/1 -> Math Function1/1
  Product/1 -> Approximation/1
  Weights/1 -> Math Function2/1
  Math Function/1 -> Regressor/1, Product/2

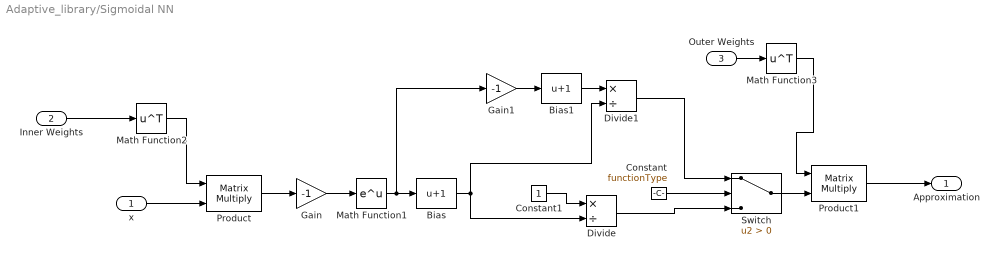
== system Adaptive_library/Sigmoidal NN ==
  x : Inport
  Inner Weights : Inport  Port=2
  Outer Weights : Inport  Port=3
  Bias : Bias  Bias=1
  Bias1 : Bias  Bias=1
  Constant : Constant  Value=functionType
  Constant1 : Constant
  Divide : Product  Inputs=*/
  Divide1 : Product  Inputs=*/
  Gain : Gain  Gain=-1
  Gain1 : Gain  Gain=-1
  Math Function1 : Math  SaturateOnIntegerOverflow=on
  Math Function2 : Math  Operator=transpose  SaturateOnIntegerOverflow=on
  Math Function3 : Math  Operator=transpose  SaturateOnIntegerOverflow=on
  Product : Product  Multiplication=Matrix(*)
  Product1 : Product  Multiplication=Matrix(*)
  Switch : Switch  Criteria=u2 > Threshold
  Approximation : Outport
  wires:
  Product1/1 -> Approximation/1
  Math Function3/1 -> Product1/1
  Outer Weights/1 -> Math Function3/1
  Divide1/1 -> Switch/1
  Switch/1 -> Product1/2
  Bias1/1 -> Divide1/1
  Gain1/1 -> Bias1/1
  Divide/1 -> Switch/3
  Constant1/1 -> Divide/1
  Bias/1 -> Divide/2, Divide1/2
  Math Function1/1 -> Bias/1, Gain1/1
  Gain/1 -> Math Function1/1
  x/1 -> Product/2
  Product/1 -> Gain/1
  Constant/1 -> Switch/2
  Math Function2/1 -> Product/1
  Inner Weights/1 -> Math Function2/1

== system Adaptive_library/eModification ==
  Err : Inport
  Estimate : Inport  Port=2
  Constant : Constant  Value=Pb
  Gain : Gain  Gain=sigma
  Norm : Adaptive_library/Norm  SystemSampleTime=-1
  Product1 : Product  Multiplication=Matrix(*)  RndMeth=Zero
  Product3 : Product  Multiplication=Matrix(*)  RndMeth=Zero
  Reshape5 : Reshape  OutputDimensionality=Row vector (2-D)
  eModification : Outport
  wires:
  Gain/1 -> eModification/1
  Err/1 -> Reshape5/1
  Constant/1 -> Product3/2
  Reshape5/1 -> Product3/1
  Estimate/1 -> Product1/1
  Product1/1 -> Gain/1
  Product3/1 -> Norm/1
  Norm/1 -> Product1/2

== system Adaptive_library/Covariance Adaptive Gain/Subsystem ==
  Gamma : Inport
  Bias : Bias  Bias=1
  Constant : Constant  Value=-Kalpha1
  Divide : Product  Inputs=*/
  Interpreted MATLAB Function : MATLABFcn  MATLABFcn=norm(u,inf)
  Product : Product  Multiplication=Matrix(*)
  alpha10 : Gain  Gain=alpha1
  alpha1*Gamma : Outport
  wires:
  Interpreted MATLAB Function/1 -> Divide/1
  Gamma/1 -> Product/2, Interpreted MATLAB Function/1
  Bias/1 -> alpha10/1
  Divide/1 -> Bias/1
  Constant/1 -> Divide/2
  alpha10/1 -> Product/1
  Product/1 -> alpha1*Gamma/1
